simulink model "simple_model"  (R2015b)
settings: Solver=ode5  StartTime=0.0  StopTime=inf  FixedStep=0.01  RelTol=1e-3
libraries: slctrlblks x1
settings Model: Creator=root  LastModifiedBy=root

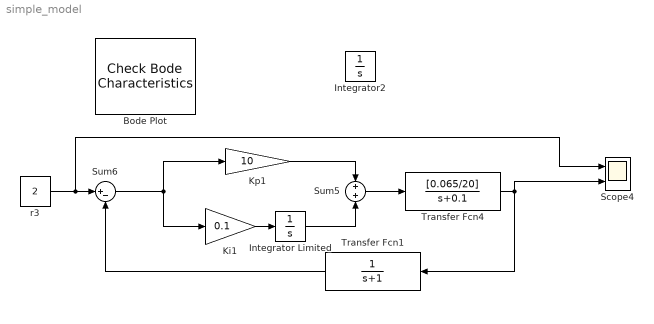
== system simple_model ==
  Bode Plot : slctrlblks/Model Verification/Check Bode  Characteristics  InstantiateOnLoad=on  SaveOperatingPoints=off  LinearizationIOs={'/Sum6', 1, 'in', 'on', '';'/Transfer Fcn1', 1, 'out', 'on', ''}  LinearizeAt=SnapshotTimes  SnapshotTimes=[0]  TriggerType=rising  SampleTime=0.0001  RateConversionMethod=zoh  PreWarpFreq=10  UseExactDelayModel=off  UseFullBlockNameLabels=off  UseBusSignalLabels=off  enabled=on  stopWhenAssertionFail=off  export=off  ViewDlgPos=[833 1 767 793]  OpenViewOnLoad=on  LaunchViewOnOpen=on  FrequencyUnits=rad/s  MagnitudeUnits=dB  PhaseUnits=deg  TimeUnits=seconds  EnableUpperBound=off  UpperBoundFrequencies=[]  UpperBoundMagnitudes=[]  EnableLowerBound=off  LowerBoundFrequencies=[]  LowerBoundMagnitudes=[]
      settings: SaveToWorkspace=on  SaveName=sys2
  Integrator Limited : Integrator  LimitOutput=on  UpperSaturationLimit=1000  LowerSaturationLimit=-1000
  Integrator2 : Integrator
  Ki1 : Gain  Gain=0.1
  Kp1 : Gain  Gain=10
  Scope4 : Scope  NumInputPorts=2
  Sum5 : Sum  Inputs=+|+
  Sum6 : Sum  Inputs=|+-
  Transfer Fcn1 : TransferFcn  Denominator=[1 1]
  Transfer Fcn4 : TransferFcn  Numerator=[0.065/20]  Denominator=[1 0.1]
  r3 : Constant  Value=2
  wires:
  Ki1/1 -> Integrator Limited/1
  Kp1/1 -> Sum5/1
  Integrator Limited/1 -> Sum5/2
  Sum6/1 -> Kp1/1, Ki1/1
  Sum5/1 -> Transfer Fcn4/1
  r3/1 -> Scope4/1, Sum6/1
  Transfer Fcn4/1 -> Transfer Fcn1/1, Scope4/2
  Transfer Fcn1/1 -> Sum6/2
